simulink model "Lab2"  (R2023a)
settings: Solver=VariableStepAuto  StartTime=0.0  StopTime=10.0  RelTol=1e-3
settings Model: Creator=Lenovo  LastModifiedBy=Lenovo

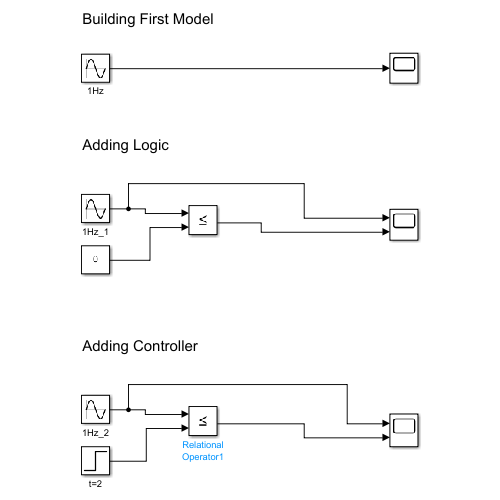
[thumbnail: Simulink's stored preview of the top-level diagram]
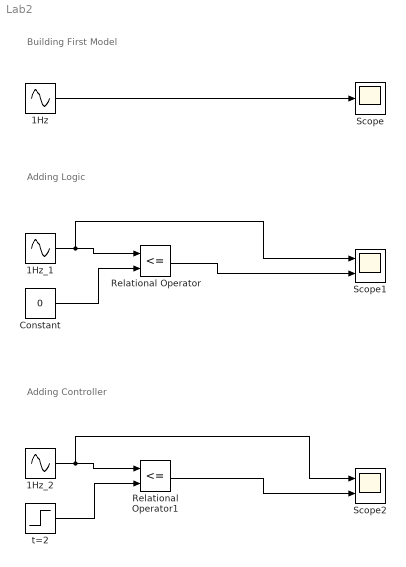
== system Lab2 ==
  note: Building First Model
  note: Adding Logic
  note: Adding Controller
  1Hz : Sin  Frequency=2*pi*1  SampleTime=0
  1Hz_1 : Sin  Frequency=2*pi*1  SampleTime=0
  1Hz_2 : Sin  Frequency=2*pi*1  SampleTime=0
  Constant : Constant  Value=0
  Relational Operator : RelationalOperator  Operator=<=  OutDataTypeStr=boolean  RndMeth=Simplest  InputSameDT=off
  Relational Operator1 : RelationalOperator  Operator=<=  OutDataTypeStr=boolean  RndMeth=Simplest  InputSameDT=off
  Scope : Scope
  Scope1 : Scope  NumInputPorts=2
  Scope2 : Scope  NumInputPorts=2
  t=2 : Step  Time=2  SampleTime=0
  wires:
  1Hz/1 -> Scope/1
  1Hz_1/1 -> Scope1/1, Relational Operator/1
  Constant/1 -> Relational Operator/2
  Relational Operator/1 -> Scope1/2
  1Hz_2/1 -> Scope2/1, Relational Operator1/1
  Relational Operator1/1 -> Scope2/2
  t=2/1 -> Relational Operator1/2
